simulink model "KD2BD_Pacsat_Modem"  (R2013a)
settings: Solver=VariableStepDiscrete  StartTime=0.0  StopTime=0.06  RelTol=1e-3
undefined symbols (not defined in the file): DiscIntNeverNeededParam
libraries: dsparch4 x3, simulink x2, simulink_extras x2, commsynccomp2 x1, commutil2 x1, commrandsrc2 x1
settings Model: Creator=tibbs2010  LastModifiedBy=Cedric

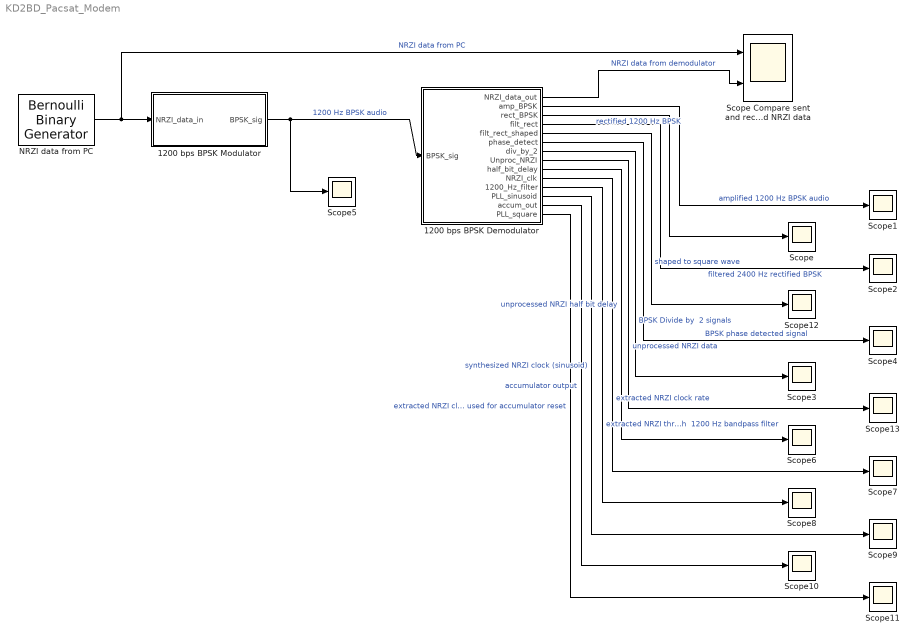
== system KD2BD_Pacsat_Modem ==
  1200 bps BPSK Demodulator : Subsystem
  1200 bps BPSK Modulator : Subsystem
  NRZI data from PC : commrandsrc2/Bernoulli Binary Generator  P=0.5  seed=61  Ts=1/1200  frameBased=off  sampPerFrame=1  orient=on  outDataType=double
  Scope{,1..13} (14 alike) : Scope
      Scope1 settings: SaveName=ScopeData2
      Scope10 settings: SaveName=ScopeData11
      Scope11 settings: SaveName=ScopeData12
      Scope12 settings: SaveName=ScopeData13
      Scope13 settings: SaveName=ScopeData14
      Scope2 settings: SaveName=ScopeData3
      Scope3 settings: SaveName=ScopeData4
      Scope4 settings: SaveName=ScopeData5
      Scope5 settings: SaveName=ScopeData6
      Scope6 settings: SaveName=ScopeData7
      Scope7 settings: SaveName=ScopeData8
      Scope8 settings: SaveName=ScopeData9
      Scope9 settings: SaveName=ScopeData10
  Scope Compare sent and received NRZI data : Scope  NumInputPorts=2
      settings: TickLabels=on  ShowLegends=on  YMin=-5~-5  YMax=5~5  MaxDataPoints=50000  SampleTime=1/(2400*100)
  wires:
  NRZI data from PC/1 -> Scope Compare sent and received NRZI data/1, 1200 bps BPSK Modulator/1(NRZI_data_in)  "NRZI data from PC"
  1200 bps BPSK Modulator/1(BPSK_sig) -> Scope5/1, 1200 bps BPSK Demodulator/1(BPSK_sig)  "1200 Hz BPSK audio"
  1200 bps BPSK Demodulator/1(NRZI_data_out) -> Scope Compare sent and received NRZI data/2  "NRZI data from demodulator"
  1200 bps BPSK Demodulator/4(filt_rect) -> Scope2/1  "filtered 2400 Hz rectified BPSK"
  1200 bps BPSK Demodulator/7(div_by_2) -> Scope3/1  "BPSK Divide by  2 signals"
  1200 bps BPSK Demodulator/6(phase_detect) -> Scope4/1  "BPSK phase detected signal"
  1200 bps BPSK Demodulator/2(amp_BPSK) -> Scope1/1  "amplified 1200 Hz BPSK audio"
  1200 bps BPSK Demodulator/3(rect_BPSK) -> Scope/1  "rectified 1200 Hz BPSK"
  1200 bps BPSK Demodulator/9(half_bit_delay) -> Scope6/1  "unprocessed NRZI half bit delay"
  1200 bps BPSK Demodulator/10(NRZI_clk) -> Scope7/1  "extracted NRZI clock rate"
  1200 bps BPSK Demodulator/11(1200_Hz_filter) -> Scope8/1  "extracted NRZI through  1200 Hz bandpass filter"
  1200 bps BPSK Demodulator/12(PLL_sinusoid) -> Scope9/1  "synthesized NRZI clock (sinusoid)"
  1200 bps BPSK Demodulator/13(accum_out) -> Scope10/1  "accumulator output"
  1200 bps BPSK Demodulator/14(PLL_square) -> Scope11/1  "extracted NRZI clock used for accumulator reset"
  1200 bps BPSK Demodulator/5(filt_rect_shaped) -> Scope12/1  "shaped to square wave"
  1200 bps BPSK Demodulator/8(Unproc_NRZI) -> Scope13/1  "unprocessed NRZI data"

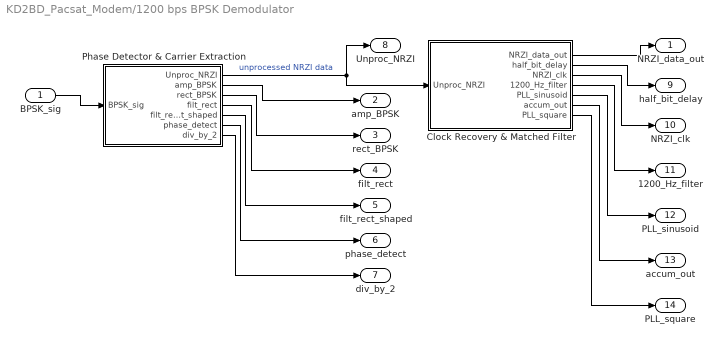
== system KD2BD_Pacsat_Modem/1200 bps BPSK Demodulator ==
  BPSK_sig : Inport
  Clock Recovery & Matched Filter : Subsystem
  Phase Detector & Carrier Extraction : Subsystem
  NRZI_data_out : Outport
  amp_BPSK : Outport  Port=2
  rect_BPSK : Outport  Port=3
  filt_rect : Outport  Port=4
  filt_rect_shaped : Outport  Port=5
  phase_detect : Outport  Port=6
  div_by_2 : Outport  Port=7
  Unproc_NRZI : Outport  Port=8
  half_bit_delay : Outport  Port=9
  NRZI_clk : Outport  Port=10
  1200_Hz_filter : Outport  Port=11
  PLL_sinusoid : Outport  Port=12
  accum_out : Outport  Port=13
  PLL_square : Outport  Port=14
  wires:
  BPSK_sig/1 -> Phase Detector & Carrier Extraction/1(BPSK_sig)
  Phase Detector & Carrier Extraction/1(Unproc_NRZI) -> Clock Recovery & Matched Filter/1(Unproc_NRZI), Unproc_NRZI/1  "unprocessed NRZI data"
  Clock Recovery & Matched Filter/1(NRZI_data_out) -> NRZI_data_out/1
  Phase Detector & Carrier Extraction/2("amp_BPSK ") -> amp_BPSK/1
  Phase Detector & Carrier Extraction/3(rect_BPSK) -> rect_BPSK/1
  Phase Detector & Carrier Extraction/4(filt_rect) -> filt_rect/1
  Phase Detector & Carrier Extraction/7(div_by_2) -> div_by_2/1
  Phase Detector & Carrier Extraction/6(phase_detect) -> phase_detect/1
  Clock Recovery & Matched Filter/2(half_bit_delay) -> half_bit_delay/1
  Clock Recovery & Matched Filter/3(NRZI_clk) -> NRZI_clk/1
  Clock Recovery & Matched Filter/4(1200_Hz_filter) -> 1200_Hz_filter/1
  Clock Recovery & Matched Filter/5(PLL_sinusoid) -> PLL_sinusoid/1
  Clock Recovery & Matched Filter/6(accum_out) -> accum_out/1
  Clock Recovery & Matched Filter/7(PLL_square) -> PLL_square/1
  Phase Detector & Carrier Extraction/5(filt_rect_shaped) -> filt_rect_shaped/1

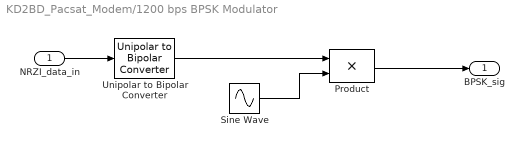
== system KD2BD_Pacsat_Modem/1200 bps BPSK Modulator ==
  NRZI_data_in : Inport
  Product : Product  SampleTime=1/(1200*100)  SaturateOnIntegerOverflow=on  OutDataTypeStr=Inherit: Same as first input
  Sine Wave : Sin  Frequency=1200*2*pi  Phase=pi/2  Samples=2400  SampleTime=1/(1200*100)
  Unipolar to Bipolar Converter : commutil2/Unipolar to Bipolar Converter  M=2  polarity=Positive  dataType=Same as input
  BPSK_sig : Outport
  wires:
  NRZI_data_in/1 -> Unipolar to Bipolar Converter/1
  Sine Wave/1 -> Product/2
  Product/1 -> BPSK_sig/1
  Unipolar to Bipolar Converter/1 -> Product/1

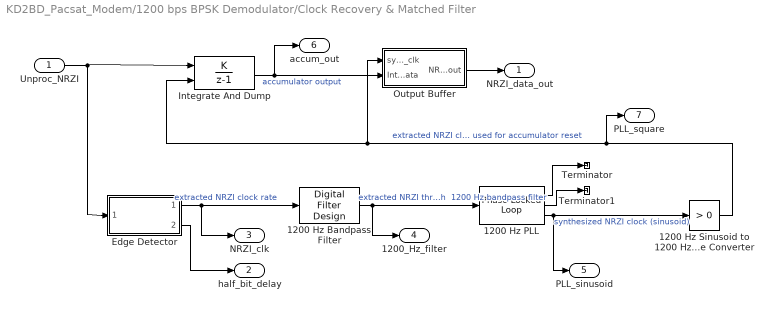
== system KD2BD_Pacsat_Modem/1200 bps BPSK Demodulator/Clock Recovery & Matched Filter ==
  Unproc_NRZI : Inport
  "1200 Hz Bandpass Filter " : dsparch4/Digital Filter Design  mwdsp_browser_bugfix_var=off
      link override Digital Filter: IIRFiltStruct=Direct form II  BiQuadCoeffs=[1 0 -1 1 -1.9600477426240257 0.98484031306811637;1 0 -1 1 -1.9657672498262708 0.98621889731216295]  ScaleValues=[0.010232556531530835;0.010232556531530835;1]  optimizeScaleValues=on
  1200 Hz PLL : commsynccomp2/Phase-Locked Loop  Fn="[3.0002  0  40002]"  Fd="[1   67.46   2270.9   40002]"  Kvco=1  Fc=1200  Ph=3.14  Ac=1
  1200 Hz Sinusoid to 1200 Hz Square Wave Converter : simulink/Logic and Bit Operations/Compare To Zero  relop=>  OutDataTypeStr=boolean
  Edge Detector : Subsystem
  Integrate And Dump : DiscreteIntegrator  IntegratorMethod=Accumulation: Forward Euler  ExternalReset=rising  InitialCondition=1  SampleTime=1/(1200*100)  ICPrevOutput=DiscIntNeverNeededParam  ICPrevScaledInput=DiscIntNeverNeededParam
  Output Buffer : Subsystem
  Terminator : Terminator
  Terminator1 : Terminator
  NRZI_data_out : Outport
  half_bit_delay : Outport  Port=2
  NRZI_clk : Outport  Port=3
  1200_Hz_filter : Outport  Port=4
  PLL_sinusoid : Outport  Port=5
  accum_out : Outport  Port=6
  PLL_square : Outport  Port=7
  wires:
  1200 Hz PLL/3 -> PLL_sinusoid/1, 1200 Hz Sinusoid to 1200 Hz Square Wave Converter/1  "synthesized NRZI clock (sinusoid)"
  1200 Hz PLL/1 -> Terminator/1
  1200 Hz PLL/2 -> Terminator1/1
  "1200 Hz Bandpass Filter "/1 -> 1200_Hz_filter/1, 1200 Hz PLL/1  "extracted NRZI through  1200 Hz bandpass filter"
  Edge Detector/1(" NRZI_clk") -> NRZI_clk/1, "1200 Hz Bandpass Filter "/1  "extracted NRZI clock rate"
  Unproc_NRZI/1 -> Edge Detector/1(Unproc_NRZI), Integrate And Dump/1
  1200 Hz Sinusoid to 1200 Hz Square Wave Converter/1 -> PLL_square/1, Integrate And Dump/2, Output Buffer/1(synth_NRZI_clk)  "extracted NRZI clock used for accumulator reset"
  Integrate And Dump/1 -> accum_out/1, Output Buffer/2(Integr_data)  "accumulator output"
  Output Buffer/1(NRZI_data_out) -> NRZI_data_out/1
  Edge Detector/2(" half_bit_delay") -> half_bit_delay/1

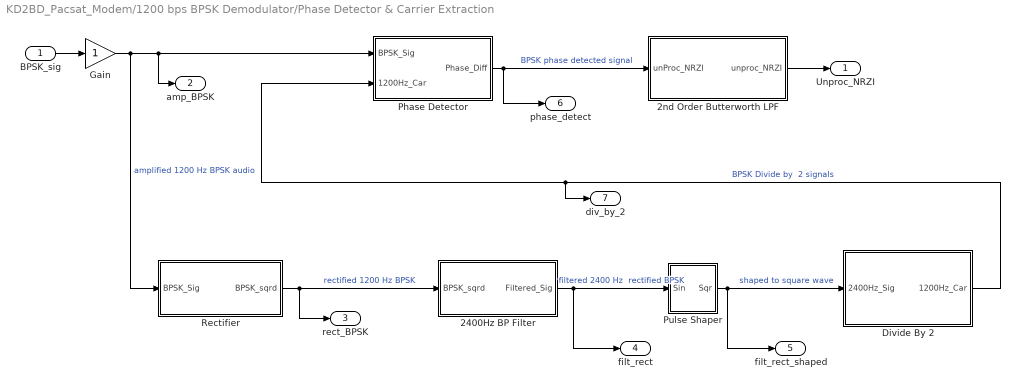
== system KD2BD_Pacsat_Modem/1200 bps BPSK Demodulator/Phase Detector & Carrier Extraction ==
  BPSK_sig : Inport
  2400Hz BP Filter : Subsystem
  "2nd Order Butterworth LPF " : Subsystem
  Divide By 2 : Subsystem
  Gain : Gain
  Phase Detector : Subsystem
  Pulse Shaper : Subsystem
  Rectifier : Subsystem
  Unproc_NRZI : Outport
  "amp_BPSK " : Outport  Port=2
  rect_BPSK : Outport  Port=3
  filt_rect : Outport  Port=4
  filt_rect_shaped : Outport  Port=5
  phase_detect : Outport  Port=6
  div_by_2 : Outport  Port=7
  wires:
  BPSK_sig/1 -> Gain/1
  Rectifier/1(BPSK_sqrd) -> rect_BPSK/1, 2400Hz BP Filter/1(BPSK_sqrd)  "rectified 1200 Hz BPSK"
  Pulse Shaper/1(Sqr) -> filt_rect_shaped/1, Divide By 2/1(2400Hz_Sig)  "shaped to square wave"
  Gain/1 -> "amp_BPSK "/1, Phase Detector/1(BPSK_Sig), Rectifier/1(BPSK_Sig)  "amplified 1200 Hz BPSK audio"
  Divide By 2/1(1200Hz_Car) -> div_by_2/1, Phase Detector/2(1200Hz_Car)  "BPSK Divide by  2 signals"
  2400Hz BP Filter/1(Filtered_Sig) -> filt_rect/1, Pulse Shaper/1(Sin)  "filtered 2400 Hz  rectified BPSK"
  Phase Detector/1(Phase_Diff) -> phase_detect/1, "2nd Order Butterworth LPF "/1(unProc_NRZI)  "BPSK phase detected signal"
  "2nd Order Butterworth LPF "/1(unproc_NRZI) -> Unproc_NRZI/1

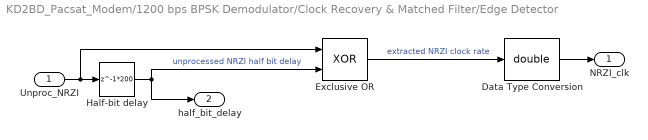
== system KD2BD_Pacsat_Modem/1200 bps BPSK Demodulator/Clock Recovery & Matched Filter/Edge Detector ==
  Unproc_NRZI : Inport
  Data Type Conversion : DataTypeConversion  OutDataTypeStr=double  SampleTime=1/(2400*200)  SaturateOnIntegerOverflow=on  RndMeth=Zero
  Exclusive OR : Logic  Operator=XOR  IconShape=distinctive  AllPortsSameDT=off  OutDataTypeStr=fixdt('boolean', 'DataTypeOverride', 'Off')
  Half-bit delay : Delay  DelayLength=1*200  InitialCondition=0  SampleTime=1/(2400*200)
  " NRZI_clk" : Outport
  " half_bit_delay" : Outport  Port=2
  wires:
  Exclusive OR/1 -> Data Type Conversion/1  "extracted NRZI clock rate"
  Half-bit delay/1 -> Exclusive OR/2, " half_bit_delay"/1  "unprocessed NRZI half bit delay"
  Data Type Conversion/1 -> " NRZI_clk"/1
  Unproc_NRZI/1 -> Exclusive OR/1, Half-bit delay/1

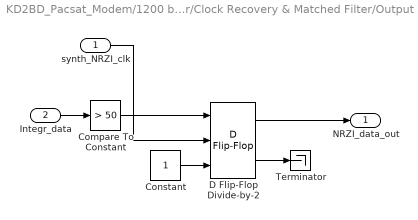
== system KD2BD_Pacsat_Modem/1200 bps BPSK Demodulator/Clock Recovery & Matched Filter/Output Buffer ==
  synth_NRZI_clk : Inport
  Integr_data : Inport  Port=2
  Compare To Constant : simulink/Logic and Bit Operations/Compare To Constant  relop=>  const=50  OutDataTypeStr=boolean
  Constant : Constant
  D Flip-Flop Divide-by-2 : simulink_extras/Flip Flops/D Flip-Flop
  Terminator : Terminator
  NRZI_data_out : Outport
  wires:
  Integr_data/1 -> Compare To Constant/1
  Compare To Constant/1 -> D Flip-Flop Divide-by-2/1
  synth_NRZI_clk/1 -> D Flip-Flop Divide-by-2/2
  D Flip-Flop Divide-by-2/1 -> NRZI_data_out/1
  Constant/1 -> D Flip-Flop Divide-by-2/3
  D Flip-Flop Divide-by-2/2 -> Terminator/1

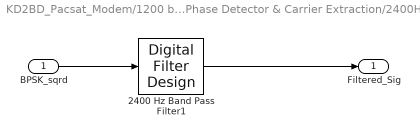
== system KD2BD_Pacsat_Modem/1200 bps BPSK Demodulator/Phase Detector & Carrier Extraction/2400Hz BP Filter ==
  BPSK_sqrd : Inport
  2400 Hz Band Pass Filter1 : dsparch4/Digital Filter Design  mwdsp_browser_bugfix_var=off
  Filtered_Sig : Outport
  wires:
  2400 Hz Band Pass Filter1/1 -> Filtered_Sig/1
  BPSK_sqrd/1 -> 2400 Hz Band Pass Filter1/1

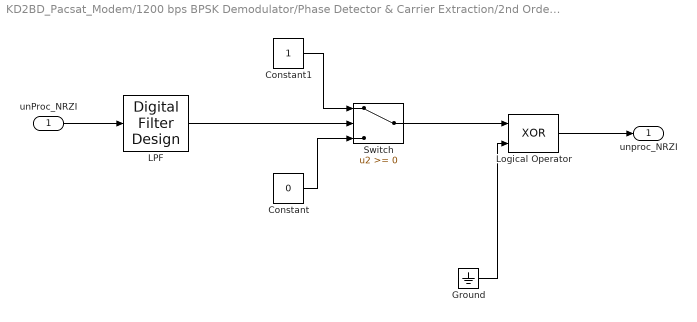
== system KD2BD_Pacsat_Modem/1200 bps BPSK Demodulator/Phase Detector & Carrier Extraction/2nd Order Butterworth LPF  ==
  unProc_NRZI : Inport
  Constant : Constant  Value=0
  Constant1 : Constant
  Ground : Ground
  LPF : dsparch4/Digital Filter Design  mwdsp_browser_bugfix_var=off
  Logical Operator : Logic  Operator=XOR  IconShape=distinctive  AllPortsSameDT=off  OutDataTypeStr=boolean
  Switch : Switch
  unproc_NRZI : Outport
  wires:
  LPF/1 -> Switch/2
  unProc_NRZI/1 -> LPF/1
  Constant/1 -> Switch/3
  Switch/1 -> Logical Operator/1
  Constant1/1 -> Switch/1
  Ground/1 -> Logical Operator/2
  Logical Operator/1 -> unproc_NRZI/1

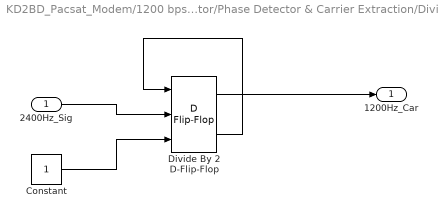
== system KD2BD_Pacsat_Modem/1200 bps BPSK Demodulator/Phase Detector & Carrier Extraction/Divide By 2 ==
  2400Hz_Sig : Inport
  Constant : Constant
  Divide By 2 D-Flip-Flop : simulink_extras/Flip Flops/D Flip-Flop
  1200Hz_Car : Outport
  wires:
  Divide By 2 D-Flip-Flop/2 -> Divide By 2 D-Flip-Flop/1
  2400Hz_Sig/1 -> Divide By 2 D-Flip-Flop/2
  Divide By 2 D-Flip-Flop/1 -> 1200Hz_Car/1
  Constant/1 -> Divide By 2 D-Flip-Flop/3

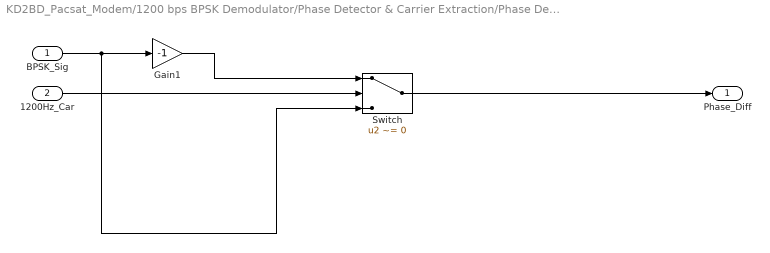
== system KD2BD_Pacsat_Modem/1200 bps BPSK Demodulator/Phase Detector & Carrier Extraction/Phase Detector ==
  BPSK_Sig : Inport
  1200Hz_Car : Inport  Port=2
  Gain1 : Gain  Gain=-1
  Switch : Switch  Criteria=u2 ~= 0  ZeroCross=off  SampleTime=1/(1200*50)
  Phase_Diff : Outport
  wires:
  1200Hz_Car/1 -> Switch/2
  BPSK_Sig/1 -> Switch/3, Gain1/1
  Switch/1 -> Phase_Diff/1
  Gain1/1 -> Switch/1

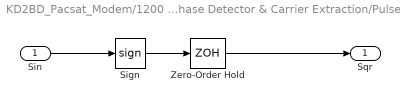
== system KD2BD_Pacsat_Modem/1200 bps BPSK Demodulator/Phase Detector & Carrier Extraction/Pulse Shaper ==
  Sin : Inport
  Sign : Signum
  Zero-Order Hold : ZeroOrderHold  SampleTime=-1
  Sqr : Outport
  wires:
  Zero-Order Hold/1 -> Sqr/1
  Sign/1 -> Zero-Order Hold/1
  Sin/1 -> Sign/1

== system KD2BD_Pacsat_Modem/1200 bps BPSK Demodulator/Phase Detector & Carrier Extraction/Rectifier ==
  BPSK_Sig : Inport
  Product : Product
  BPSK_sqrd : Outport
  wires:
  BPSK_Sig/1 -> Product/1, Product/2
  Product/1 -> BPSK_sqrd/1
